simulink model "LV_grid"  (R2021b)
settings: Solver=VariableStepAuto  StartTime=0  StopTime=5.0005  FixedStep=5e-4  RelTol=1e-3
model workspace (MAT data in the model file):
  P2_1 = 3450
  idx = 1
  time_counter = 1
libraries: spsGroundLib x97, spsStairGeneratorLib x96, spsPiSectionLineLib x90, spsThreePhasePISectionLineLib x90, spsVariableInductorLib x48, spsVariableResistorLib x48, spsRMSLib x36, spsThreePhaseVIMeasurementLib x34, spsACVoltageSourceLib x5, spsLinearTransformerLib x5, spsPower3phInstantaneousLib x1, spsThreePhaseMutualInductanceZ1Z0Lib x1
(part 2 of 6)

== system LV_grid/B16 ==
  MATLAB Function : MATLAB Function  TreatAsAtomicUnit=on
  RMS : spsRMSLib/RMS  TrueRMS=on  Freq=50  RMSInit=1  Ts=5e-4
  Three-Phase V-I Measurement : spsThreePhaseVIMeasurementLib/Three-Phase V-I Measurement  VoltageMeasurement=phase-to-ground  SetLabelV=off  LabelV=Vabc_B1  Vpu=on  VpuLL=off  CurrentMeasurement=no  SetLabelI=off  LabelI=Iabc  Ipu=off  Pbase=100e6  Vbase=400/sqrt(2)  OutputType=Complex  PhasorSimulation=off  PSBequivalent=0
  A : PMIOPort  Side=Left
  B : PMIOPort  Port=2  Side=Left
  C : PMIOPort  Port=3  Side=Left
  "N " : PMIOPort  Tag=PMCPort  Port=4  Side=Left
  a : PMIOPort  Tag=PMCPort  Port=5  Side=Right
  b : PMIOPort  Tag=PMCPort  Port=6  Side=Right
  c : PMIOPort  Tag=PMCPort  Port=7  Side=Right
  n : PMIOPort  Tag=PMCPort  Port=8  Side=Right
  V_out : Outport
  tag scope: Vabc_B16=global
  wires:
  Three-Phase V-I Measurement/1 -> RMS/1
  RMS/1 -> MATLAB Function/1(u)
  MATLAB Function/1(y) -> [Vabc_B16], V_out/1
  connections:
  A/RConn1 -- Three-Phase V-I Measurement/LConn1
  B/RConn1 -- Three-Phase V-I Measurement/LConn2
  C/RConn1 -- Three-Phase V-I Measurement/LConn3
  a/RConn1 -- Three-Phase V-I Measurement/RConn1
  b/RConn1 -- Three-Phase V-I Measurement/RConn2
  c/RConn1 -- Three-Phase V-I Measurement/RConn3
  n/RConn1 -- "N "/RConn1

== system LV_grid/B17 ==
  MATLAB Function : MATLAB Function  TreatAsAtomicUnit=on
  RMS : spsRMSLib/RMS  TrueRMS=on  Freq=50  RMSInit=1  Ts=5e-4
  Three-Phase V-I Measurement : spsThreePhaseVIMeasurementLib/Three-Phase V-I Measurement  VoltageMeasurement=phase-to-ground  SetLabelV=off  LabelV=Vabc_B1  Vpu=on  VpuLL=off  CurrentMeasurement=no  SetLabelI=off  LabelI=Iabc  Ipu=off  Pbase=100e6  Vbase=400/sqrt(2)  OutputType=Complex  PhasorSimulation=off  PSBequivalent=0
  A : PMIOPort  Side=Left
  B : PMIOPort  Port=2  Side=Left
  C : PMIOPort  Port=3  Side=Left
  "N " : PMIOPort  Tag=PMCPort  Port=4  Side=Left
  a : PMIOPort  Tag=PMCPort  Port=5  Side=Right
  b : PMIOPort  Tag=PMCPort  Port=6  Side=Right
  c : PMIOPort  Tag=PMCPort  Port=7  Side=Right
  n : PMIOPort  Tag=PMCPort  Port=8  Side=Right
  V_out : Outport
  tag scope: Vabc_B17=global
  wires:
  Three-Phase V-I Measurement/1 -> RMS/1
  RMS/1 -> MATLAB Function/1(u)
  MATLAB Function/1(y) -> [Vabc_B17], V_out/1
  connections:
  A/RConn1 -- Three-Phase V-I Measurement/LConn1
  B/RConn1 -- Three-Phase V-I Measurement/LConn2
  C/RConn1 -- Three-Phase V-I Measurement/LConn3
  a/RConn1 -- Three-Phase V-I Measurement/RConn1
  b/RConn1 -- Three-Phase V-I Measurement/RConn2
  c/RConn1 -- Three-Phase V-I Measurement/RConn3
  n/RConn1 -- "N "/RConn1

== system LV_grid/B18 ==
  MATLAB Function : MATLAB Function  TreatAsAtomicUnit=on
  RMS : spsRMSLib/RMS  TrueRMS=on  Freq=50  RMSInit=1  Ts=5e-4
  Three-Phase V-I Measurement : spsThreePhaseVIMeasurementLib/Three-Phase V-I Measurement  VoltageMeasurement=phase-to-ground  SetLabelV=off  LabelV=Vabc_B1  Vpu=on  VpuLL=off  CurrentMeasurement=no  SetLabelI=off  LabelI=Iabc  Ipu=off  Pbase=100e6  Vbase=400/sqrt(2)  OutputType=Complex  PhasorSimulation=off  PSBequivalent=0
  A : PMIOPort  Side=Left
  B : PMIOPort  Port=2  Side=Left
  C : PMIOPort  Port=3  Side=Left
  "N " : PMIOPort  Tag=PMCPort  Port=4  Side=Left
  a : PMIOPort  Tag=PMCPort  Port=5  Side=Right
  b : PMIOPort  Tag=PMCPort  Port=6  Side=Right
  c : PMIOPort  Tag=PMCPort  Port=7  Side=Right
  n : PMIOPort  Tag=PMCPort  Port=8  Side=Right
  V_out : Outport
  tag scope: Vabc_B18=global
  wires:
  Three-Phase V-I Measurement/1 -> RMS/1
  RMS/1 -> MATLAB Function/1(u)
  MATLAB Function/1(y) -> [Vabc_B18], V_out/1
  connections:
  A/RConn1 -- Three-Phase V-I Measurement/LConn1
  B/RConn1 -- Three-Phase V-I Measurement/LConn2
  C/RConn1 -- Three-Phase V-I Measurement/LConn3
  a/RConn1 -- Three-Phase V-I Measurement/RConn1
  b/RConn1 -- Three-Phase V-I Measurement/RConn2
  c/RConn1 -- Three-Phase V-I Measurement/RConn3
  n/RConn1 -- "N "/RConn1

== system LV_grid/B19 ==
  MATLAB Function : MATLAB Function  TreatAsAtomicUnit=on
  RMS : spsRMSLib/RMS  TrueRMS=on  Freq=50  RMSInit=1  Ts=5e-4
  Three-Phase V-I Measurement : spsThreePhaseVIMeasurementLib/Three-Phase V-I Measurement  VoltageMeasurement=phase-to-ground  SetLabelV=off  LabelV=Vabc_B1  Vpu=on  VpuLL=off  CurrentMeasurement=no  SetLabelI=off  LabelI=Iabc  Ipu=off  Pbase=100e6  Vbase=400/sqrt(2)  OutputType=Complex  PhasorSimulation=off  PSBequivalent=0
  A : PMIOPort  Side=Left
  B : PMIOPort  Port=2  Side=Left
  C : PMIOPort  Port=3  Side=Left
  "N " : PMIOPort  Tag=PMCPort  Port=4  Side=Left
  a : PMIOPort  Tag=PMCPort  Port=5  Side=Right
  b : PMIOPort  Tag=PMCPort  Port=6  Side=Right
  c : PMIOPort  Tag=PMCPort  Port=7  Side=Right
  n : PMIOPort  Tag=PMCPort  Port=8  Side=Right
  V_out : Outport
  tag scope: Vabc_B19=global
  wires:
  Three-Phase V-I Measurement/1 -> RMS/1
  MATLAB Function/1(y) -> [Vabc_B19], V_out/1
  RMS/1 -> MATLAB Function/1(u)
  connections:
  A/RConn1 -- Three-Phase V-I Measurement/LConn1
  B/RConn1 -- Three-Phase V-I Measurement/LConn2
  C/RConn1 -- Three-Phase V-I Measurement/LConn3
  a/RConn1 -- Three-Phase V-I Measurement/RConn1
  b/RConn1 -- Three-Phase V-I Measurement/RConn2
  c/RConn1 -- Three-Phase V-I Measurement/RConn3
  n/RConn1 -- "N "/RConn1

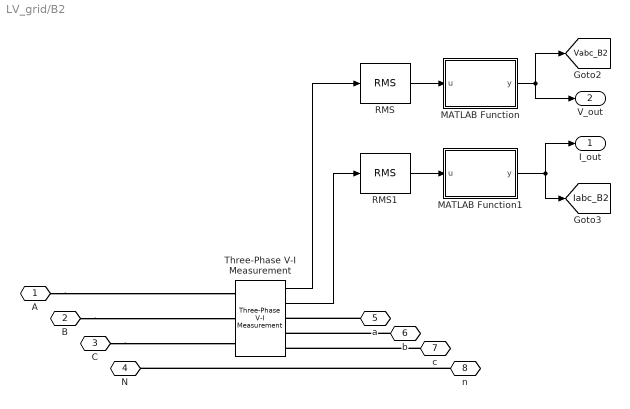
== system LV_grid/B2 ==
  MATLAB Function : MATLAB Function  TreatAsAtomicUnit=on
  MATLAB Function1 : MATLAB Function  TreatAsAtomicUnit=on
  RMS : spsRMSLib/RMS  TrueRMS=on  Freq=50  RMSInit=1  Ts=5e-4
  RMS1 : spsRMSLib/RMS  TrueRMS=on  Freq=50  RMSInit=1  Ts=5e-4
  Three-Phase V-I Measurement : spsThreePhaseVIMeasurementLib/Three-Phase V-I Measurement  VoltageMeasurement=phase-to-ground  SetLabelV=off  LabelV=Vabc_B1  Vpu=on  VpuLL=off  CurrentMeasurement=yes  SetLabelI=off  LabelI=Iabc  Ipu=on  Pbase=250e3  Vbase=400/sqrt(2)  OutputType=Magnitude  PhasorSimulation=off  PSBequivalent=0
  A : PMIOPort  Side=Left
  B : PMIOPort  Port=2  Side=Left
  C : PMIOPort  Port=3  Side=Left
  N : PMIOPort  Tag=PMCPort  Port=4  Side=Left
  a : PMIOPort  Tag=PMCPort  Port=5  Side=Right
  b : PMIOPort  Tag=PMCPort  Port=6  Side=Right
  c : PMIOPort  Tag=PMCPort  Port=7  Side=Right
  n : PMIOPort  Tag=PMCPort  Port=8  Side=Right
  I_out : Outport
  V_out : Outport  Port=2
  tag scope: Iabc_B2=global, Vabc_B2=global
  wires:
  Three-Phase V-I Measurement/1 -> RMS/1
  Three-Phase V-I Measurement/2 -> RMS1/1
  MATLAB Function/1(y) -> [Vabc_B2], V_out/1
  RMS/1 -> MATLAB Function/1(u)
  RMS1/1 -> MATLAB Function1/1(u)
  MATLAB Function1/1(y) -> [Iabc_B2], I_out/1
  connections:
  B/RConn1 -- Three-Phase V-I Measurement/LConn2
  n/RConn1 -- N/RConn1
  c/RConn1 -- Three-Phase V-I Measurement/RConn3
  b/RConn1 -- Three-Phase V-I Measurement/RConn2
  C/RConn1 -- Three-Phase V-I Measurement/LConn3
  a/RConn1 -- Three-Phase V-I Measurement/RConn1
  A/RConn1 -- Three-Phase V-I Measurement/LConn1

== system LV_grid/B20 ==
  MATLAB Function : MATLAB Function  TreatAsAtomicUnit=on
  RMS : spsRMSLib/RMS  TrueRMS=on  Freq=50  RMSInit=1  Ts=5e-4
  Three-Phase V-I Measurement : spsThreePhaseVIMeasurementLib/Three-Phase V-I Measurement  VoltageMeasurement=phase-to-ground  SetLabelV=off  LabelV=Vabc_B1  Vpu=on  VpuLL=off  CurrentMeasurement=no  SetLabelI=off  LabelI=Iabc  Ipu=off  Pbase=100e6  Vbase=400/sqrt(2)  OutputType=Complex  PhasorSimulation=off  PSBequivalent=0
  A : PMIOPort  Side=Left
  B : PMIOPort  Port=2  Side=Left
  C : PMIOPort  Port=3  Side=Left
  "N " : PMIOPort  Tag=PMCPort  Port=4  Side=Left
  a : PMIOPort  Tag=PMCPort  Port=5  Side=Right
  b : PMIOPort  Tag=PMCPort  Port=6  Side=Right
  c : PMIOPort  Tag=PMCPort  Port=7  Side=Right
  n : PMIOPort  Tag=PMCPort  Port=8  Side=Right
  V_out : Outport
  tag scope: Vabc_B20=global
  wires:
  Three-Phase V-I Measurement/1 -> RMS/1
  RMS/1 -> MATLAB Function/1(u)
  MATLAB Function/1(y) -> [Vabc_B20], V_out/1
  connections:
  A/RConn1 -- Three-Phase V-I Measurement/LConn1
  B/RConn1 -- Three-Phase V-I Measurement/LConn2
  C/RConn1 -- Three-Phase V-I Measurement/LConn3
  a/RConn1 -- Three-Phase V-I Measurement/RConn1
  b/RConn1 -- Three-Phase V-I Measurement/RConn2
  c/RConn1 -- Three-Phase V-I Measurement/RConn3
  n/RConn1 -- "N "/RConn1

== system LV_grid/B21 ==
  MATLAB Function : MATLAB Function  TreatAsAtomicUnit=on
  RMS : spsRMSLib/RMS  TrueRMS=on  Freq=50  RMSInit=1  Ts=5e-4
  Three-Phase V-I Measurement : spsThreePhaseVIMeasurementLib/Three-Phase V-I Measurement  VoltageMeasurement=phase-to-ground  SetLabelV=off  LabelV=Vabc_B1  Vpu=on  VpuLL=off  CurrentMeasurement=no  SetLabelI=off  LabelI=Iabc  Ipu=off  Pbase=100e6  Vbase=400/sqrt(2)  OutputType=Complex  PhasorSimulation=off  PSBequivalent=0
  A : PMIOPort  Side=Left
  B : PMIOPort  Port=2  Side=Left
  C : PMIOPort  Port=3  Side=Left
  "N " : PMIOPort  Tag=PMCPort  Port=4  Side=Left
  a : PMIOPort  Tag=PMCPort  Port=5  Side=Right
  b : PMIOPort  Tag=PMCPort  Port=6  Side=Right
  c : PMIOPort  Tag=PMCPort  Port=7  Side=Right
  n : PMIOPort  Tag=PMCPort  Port=8  Side=Right
  V_out : Outport
  tag scope: Vabc_B21=global
  wires:
  Three-Phase V-I Measurement/1 -> RMS/1
  RMS/1 -> MATLAB Function/1(u)
  MATLAB Function/1(y) -> [Vabc_B21], V_out/1
  connections:
  A/RConn1 -- Three-Phase V-I Measurement/LConn1
  B/RConn1 -- Three-Phase V-I Measurement/LConn2
  C/RConn1 -- Three-Phase V-I Measurement/LConn3
  a/RConn1 -- Three-Phase V-I Measurement/RConn1
  b/RConn1 -- Three-Phase V-I Measurement/RConn2
  c/RConn1 -- Three-Phase V-I Measurement/RConn3
  n/RConn1 -- "N "/RConn1

== system LV_grid/B22 ==
  MATLAB Function : MATLAB Function  TreatAsAtomicUnit=on
  RMS : spsRMSLib/RMS  TrueRMS=on  Freq=50  RMSInit=1  Ts=5e-4
  Three-Phase V-I Measurement : spsThreePhaseVIMeasurementLib/Three-Phase V-I Measurement  VoltageMeasurement=phase-to-ground  SetLabelV=off  LabelV=Vabc_B1  Vpu=on  VpuLL=off  CurrentMeasurement=no  SetLabelI=off  LabelI=Iabc  Ipu=off  Pbase=100e6  Vbase=400/sqrt(2)  OutputType=Complex  PhasorSimulation=off  PSBequivalent=0
  A : PMIOPort  Side=Left
  B : PMIOPort  Port=2  Side=Left
  C : PMIOPort  Port=3  Side=Left
  "N " : PMIOPort  Tag=PMCPort  Port=4  Side=Left
  a : PMIOPort  Tag=PMCPort  Port=5  Side=Right
  b : PMIOPort  Tag=PMCPort  Port=6  Side=Right
  c : PMIOPort  Tag=PMCPort  Port=7  Side=Right
  n : PMIOPort  Tag=PMCPort  Port=8  Side=Right
  V_out : Outport
  tag scope: Vabc_B22=global
  wires:
  Three-Phase V-I Measurement/1 -> RMS/1
  RMS/1 -> MATLAB Function/1(u)
  MATLAB Function/1(y) -> [Vabc_B22], V_out/1
  connections:
  A/RConn1 -- Three-Phase V-I Measurement/LConn1
  B/RConn1 -- Three-Phase V-I Measurement/LConn2
  C/RConn1 -- Three-Phase V-I Measurement/LConn3
  a/RConn1 -- Three-Phase V-I Measurement/RConn1
  b/RConn1 -- Three-Phase V-I Measurement/RConn2
  c/RConn1 -- Three-Phase V-I Measurement/RConn3
  n/RConn1 -- "N "/RConn1

== system LV_grid/B23 ==
  MATLAB Function : MATLAB Function  TreatAsAtomicUnit=on
  RMS : spsRMSLib/RMS  TrueRMS=on  Freq=50  RMSInit=1  Ts=5e-4
  Three-Phase V-I Measurement : spsThreePhaseVIMeasurementLib/Three-Phase V-I Measurement  VoltageMeasurement=phase-to-ground  SetLabelV=off  LabelV=Vabc_B1  Vpu=on  VpuLL=off  CurrentMeasurement=no  SetLabelI=off  LabelI=Iabc  Ipu=off  Pbase=100e6  Vbase=400/sqrt(2)  OutputType=Complex  PhasorSimulation=off  PSBequivalent=0
  A : PMIOPort  Side=Left
  B : PMIOPort  Port=2  Side=Left
  C : PMIOPort  Port=3  Side=Left
  "N " : PMIOPort  Tag=PMCPort  Port=4  Side=Left
  a : PMIOPort  Tag=PMCPort  Port=5  Side=Right
  b : PMIOPort  Tag=PMCPort  Port=6  Side=Right
  c : PMIOPort  Tag=PMCPort  Port=7  Side=Right
  n : PMIOPort  Tag=PMCPort  Port=8  Side=Right
  V_out : Outport
  tag scope: Vabc_B23=global
  wires:
  Three-Phase V-I Measurement/1 -> RMS/1
  RMS/1 -> MATLAB Function/1(u)
  MATLAB Function/1(y) -> [Vabc_B23], V_out/1
  connections:
  A/RConn1 -- Three-Phase V-I Measurement/LConn1
  B/RConn1 -- Three-Phase V-I Measurement/LConn2
  C/RConn1 -- Three-Phase V-I Measurement/LConn3
  a/RConn1 -- Three-Phase V-I Measurement/RConn1
  b/RConn1 -- Three-Phase V-I Measurement/RConn2
  c/RConn1 -- Three-Phase V-I Measurement/RConn3
  n/RConn1 -- "N "/RConn1

== system LV_grid/B24 ==
  MATLAB Function : MATLAB Function  TreatAsAtomicUnit=on
  RMS : spsRMSLib/RMS  TrueRMS=on  Freq=50  RMSInit=1  Ts=5e-4
  Three-Phase V-I Measurement : spsThreePhaseVIMeasurementLib/Three-Phase V-I Measurement  VoltageMeasurement=phase-to-ground  SetLabelV=off  LabelV=Vabc_B1  Vpu=on  VpuLL=off  CurrentMeasurement=no  SetLabelI=off  LabelI=Iabc  Ipu=off  Pbase=100e6  Vbase=400/sqrt(2)  OutputType=Complex  PhasorSimulation=off  PSBequivalent=0
  A : PMIOPort  Side=Left
  B : PMIOPort  Port=2  Side=Left
  C : PMIOPort  Port=3  Side=Left
  "N " : PMIOPort  Tag=PMCPort  Port=4  Side=Left
  a : PMIOPort  Tag=PMCPort  Port=5  Side=Right
  b : PMIOPort  Tag=PMCPort  Port=6  Side=Right
  c : PMIOPort  Tag=PMCPort  Port=7  Side=Right
  n : PMIOPort  Tag=PMCPort  Port=8  Side=Right
  V_out : Outport
  tag scope: Vabc_B24=global
  wires:
  Three-Phase V-I Measurement/1 -> RMS/1
  RMS/1 -> MATLAB Function/1(u)
  MATLAB Function/1(y) -> [Vabc_B24], V_out/1
  connections:
  A/RConn1 -- Three-Phase V-I Measurement/LConn1
  B/RConn1 -- Three-Phase V-I Measurement/LConn2
  C/RConn1 -- Three-Phase V-I Measurement/LConn3
  a/RConn1 -- Three-Phase V-I Measurement/RConn1
  b/RConn1 -- Three-Phase V-I Measurement/RConn2
  c/RConn1 -- Three-Phase V-I Measurement/RConn3
  n/RConn1 -- "N "/RConn1

== system LV_grid/B25 ==
  MATLAB Function : MATLAB Function  TreatAsAtomicUnit=on
  RMS : spsRMSLib/RMS  TrueRMS=on  Freq=50  RMSInit=1  Ts=5e-4
  Three-Phase V-I Measurement : spsThreePhaseVIMeasurementLib/Three-Phase V-I Measurement  VoltageMeasurement=phase-to-ground  SetLabelV=off  LabelV=Vabc_B1  Vpu=on  VpuLL=off  CurrentMeasurement=no  SetLabelI=off  LabelI=Iabc  Ipu=off  Pbase=100e6  Vbase=400/sqrt(2)  OutputType=Complex  PhasorSimulation=off  PSBequivalent=0
  A : PMIOPort  Side=Left
  B : PMIOPort  Port=2  Side=Left
  C : PMIOPort  Port=3  Side=Left
  "N " : PMIOPort  Tag=PMCPort  Port=4  Side=Left
  a : PMIOPort  Tag=PMCPort  Port=5  Side=Right
  b : PMIOPort  Tag=PMCPort  Port=6  Side=Right
  c : PMIOPort  Tag=PMCPort  Port=7  Side=Right
  n : PMIOPort  Tag=PMCPort  Port=8  Side=Right
  V_out : Outport
  tag scope: Vabc_B25=global
  wires:
  Three-Phase V-I Measurement/1 -> RMS/1
  RMS/1 -> MATLAB Function/1(u)
  MATLAB Function/1(y) -> [Vabc_B25], V_out/1
  connections:
  A/RConn1 -- Three-Phase V-I Measurement/LConn1
  B/RConn1 -- Three-Phase V-I Measurement/LConn2
  C/RConn1 -- Three-Phase V-I Measurement/LConn3
  a/RConn1 -- Three-Phase V-I Measurement/RConn1
  b/RConn1 -- Three-Phase V-I Measurement/RConn2
  c/RConn1 -- Three-Phase V-I Measurement/RConn3
  n/RConn1 -- "N "/RConn1

== system LV_grid/B26 ==
  MATLAB Function : MATLAB Function  TreatAsAtomicUnit=on
  RMS : spsRMSLib/RMS  TrueRMS=on  Freq=50  RMSInit=1  Ts=5e-4
  Three-Phase V-I Measurement : spsThreePhaseVIMeasurementLib/Three-Phase V-I Measurement  VoltageMeasurement=phase-to-ground  SetLabelV=off  LabelV=Vabc_B1  Vpu=on  VpuLL=off  CurrentMeasurement=no  SetLabelI=off  LabelI=Iabc  Ipu=off  Pbase=100e6  Vbase=400/sqrt(2)  OutputType=Complex  PhasorSimulation=off  PSBequivalent=0
  A : PMIOPort  Side=Left
  B : PMIOPort  Port=2  Side=Left
  C : PMIOPort  Port=3  Side=Left
  "N " : PMIOPort  Tag=PMCPort  Port=4  Side=Left
  a : PMIOPort  Tag=PMCPort  Port=5  Side=Right
  b : PMIOPort  Tag=PMCPort  Port=6  Side=Right
  c : PMIOPort  Tag=PMCPort  Port=7  Side=Right
  n : PMIOPort  Tag=PMCPort  Port=8  Side=Right
  V_out : Outport
  tag scope: Vabc_B26=global
  wires:
  Three-Phase V-I Measurement/1 -> RMS/1
  RMS/1 -> MATLAB Function/1(u)
  MATLAB Function/1(y) -> [Vabc_B26], V_out/1
  connections:
  A/RConn1 -- Three-Phase V-I Measurement/LConn1
  B/RConn1 -- Three-Phase V-I Measurement/LConn2
  C/RConn1 -- Three-Phase V-I Measurement/LConn3
  a/RConn1 -- Three-Phase V-I Measurement/RConn1
  b/RConn1 -- Three-Phase V-I Measurement/RConn2
  c/RConn1 -- Three-Phase V-I Measurement/RConn3
  n/RConn1 -- "N "/RConn1

== system LV_grid/B27 ==
  MATLAB Function : MATLAB Function  TreatAsAtomicUnit=on
  RMS : spsRMSLib/RMS  TrueRMS=on  Freq=50  RMSInit=1  Ts=5e-4
  Three-Phase V-I Measurement : spsThreePhaseVIMeasurementLib/Three-Phase V-I Measurement  VoltageMeasurement=phase-to-ground  SetLabelV=off  LabelV=Vabc_B1  Vpu=on  VpuLL=off  CurrentMeasurement=no  SetLabelI=off  LabelI=Iabc  Ipu=off  Pbase=100e6  Vbase=400/sqrt(2)  OutputType=Complex  PhasorSimulation=off  PSBequivalent=0
  A : PMIOPort  Side=Left
  B : PMIOPort  Port=2  Side=Left
  C : PMIOPort  Port=3  Side=Left
  "N " : PMIOPort  Tag=PMCPort  Port=4  Side=Left
  a : PMIOPort  Tag=PMCPort  Port=5  Side=Right
  b : PMIOPort  Tag=PMCPort  Port=6  Side=Right
  c : PMIOPort  Tag=PMCPort  Port=7  Side=Right
  n : PMIOPort  Tag=PMCPort  Port=8  Side=Right
  V_out : Outport
  tag scope: Vabc_B27=global
  wires:
  Three-Phase V-I Measurement/1 -> RMS/1
  RMS/1 -> MATLAB Function/1(u)
  MATLAB Function/1(y) -> [Vabc_B27], V_out/1
  connections:
  A/RConn1 -- Three-Phase V-I Measurement/LConn1
  B/RConn1 -- Three-Phase V-I Measurement/LConn2
  C/RConn1 -- Three-Phase V-I Measurement/LConn3
  a/RConn1 -- Three-Phase V-I Measurement/RConn1
  b/RConn1 -- Three-Phase V-I Measurement/RConn2
  c/RConn1 -- Three-Phase V-I Measurement/RConn3
  n/RConn1 -- "N "/RConn1

== system LV_grid/B28 ==
  MATLAB Function : MATLAB Function  TreatAsAtomicUnit=on
  RMS : spsRMSLib/RMS  TrueRMS=on  Freq=50  RMSInit=1  Ts=5e-4
  Three-Phase V-I Measurement : spsThreePhaseVIMeasurementLib/Three-Phase V-I Measurement  VoltageMeasurement=phase-to-ground  SetLabelV=off  LabelV=Vabc_B1  Vpu=on  VpuLL=off  CurrentMeasurement=no  SetLabelI=off  LabelI=Iabc  Ipu=off  Pbase=100e6  Vbase=400/sqrt(2)  OutputType=Complex  PhasorSimulation=off  PSBequivalent=0
  A : PMIOPort  Side=Left
  B : PMIOPort  Port=2  Side=Left
  C : PMIOPort  Port=3  Side=Left
  "N " : PMIOPort  Tag=PMCPort  Port=4  Side=Left
  a : PMIOPort  Tag=PMCPort  Port=5  Side=Right
  b : PMIOPort  Tag=PMCPort  Port=6  Side=Right
  c : PMIOPort  Tag=PMCPort  Port=7  Side=Right
  n : PMIOPort  Tag=PMCPort  Port=8  Side=Right
  V_out : Outport
  tag scope: Vabc_B28=global
  wires:
  Three-Phase V-I Measurement/1 -> RMS/1
  RMS/1 -> MATLAB Function/1(u)
  MATLAB Function/1(y) -> [Vabc_B28], V_out/1
  connections:
  A/RConn1 -- Three-Phase V-I Measurement/LConn1
  B/RConn1 -- Three-Phase V-I Measurement/LConn2
  C/RConn1 -- Three-Phase V-I Measurement/LConn3
  a/RConn1 -- Three-Phase V-I Measurement/RConn1
  b/RConn1 -- Three-Phase V-I Measurement/RConn2
  c/RConn1 -- Three-Phase V-I Measurement/RConn3
  n/RConn1 -- "N "/RConn1

== system LV_grid/B29 ==
  MATLAB Function : MATLAB Function  TreatAsAtomicUnit=on
  RMS : spsRMSLib/RMS  TrueRMS=on  Freq=50  RMSInit=1  Ts=5e-4
  Three-Phase V-I Measurement : spsThreePhaseVIMeasurementLib/Three-Phase V-I Measurement  VoltageMeasurement=phase-to-ground  SetLabelV=off  LabelV=Vabc_B1  Vpu=on  VpuLL=off  CurrentMeasurement=no  SetLabelI=off  LabelI=Iabc  Ipu=off  Pbase=100e6  Vbase=400/sqrt(2)  OutputType=Complex  PhasorSimulation=off  PSBequivalent=0
  A : PMIOPort  Side=Left
  B : PMIOPort  Port=2  Side=Left
  C : PMIOPort  Port=3  Side=Left
  "N " : PMIOPort  Tag=PMCPort  Port=4  Side=Left
  a : PMIOPort  Tag=PMCPort  Port=5  Side=Right
  b : PMIOPort  Tag=PMCPort  Port=6  Side=Right
  c : PMIOPort  Tag=PMCPort  Port=7  Side=Right
  n : PMIOPort  Tag=PMCPort  Port=8  Side=Right
  V_out : Outport
  tag scope: Vabc_B29=global
  wires:
  Three-Phase V-I Measurement/1 -> RMS/1
  RMS/1 -> MATLAB Function/1(u)
  MATLAB Function/1(y) -> [Vabc_B29], V_out/1
  connections:
  A/RConn1 -- Three-Phase V-I Measurement/LConn1
  B/RConn1 -- Three-Phase V-I Measurement/LConn2
  C/RConn1 -- Three-Phase V-I Measurement/LConn3
  a/RConn1 -- Three-Phase V-I Measurement/RConn1
  b/RConn1 -- Three-Phase V-I Measurement/RConn2
  c/RConn1 -- Three-Phase V-I Measurement/RConn3
  n/RConn1 -- "N "/RConn1

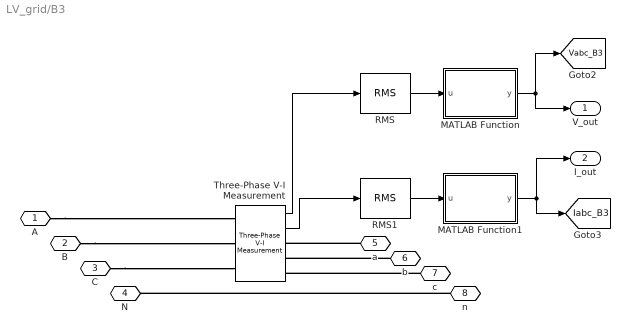
== system LV_grid/B3 ==
  MATLAB Function : MATLAB Function  TreatAsAtomicUnit=on
  MATLAB Function1 : MATLAB Function  TreatAsAtomicUnit=on
  RMS : spsRMSLib/RMS  TrueRMS=on  Freq=50  RMSInit=1  Ts=5e-4
  RMS1 : spsRMSLib/RMS  TrueRMS=on  Freq=50  RMSInit=1  Ts=5e-4
  Three-Phase V-I Measurement : spsThreePhaseVIMeasurementLib/Three-Phase V-I Measurement  VoltageMeasurement=phase-to-ground  SetLabelV=off  LabelV=Vabc_B1  Vpu=on  VpuLL=off  CurrentMeasurement=yes  SetLabelI=off  LabelI=Iabc  Ipu=on  Pbase=250e3  Vbase=400/sqrt(2)  OutputType=Magnitude  PhasorSimulation=off  PSBequivalent=0
  A : PMIOPort  Side=Left
  B : PMIOPort  Port=2  Side=Left
  C : PMIOPort  Port=3  Side=Left
  N : PMIOPort  Tag=PMCPort  Port=4  Side=Left
  a : PMIOPort  Tag=PMCPort  Port=5  Side=Right
  b : PMIOPort  Tag=PMCPort  Port=6  Side=Right
  c : PMIOPort  Tag=PMCPort  Port=7  Side=Right
  n : PMIOPort  Tag=PMCPort  Port=8  Side=Right
  V_out : Outport
  I_out : Outport  Port=2
  tag scope: Iabc_B3=global, Vabc_B3=global
  wires:
  Three-Phase V-I Measurement/2 -> RMS1/1
  RMS/1 -> MATLAB Function/1(u)
  MATLAB Function/1(y) -> V_out/1, [Vabc_B3]
  Three-Phase V-I Measurement/1 -> RMS/1
  MATLAB Function1/1(y) -> [Iabc_B3], I_out/1
  RMS1/1 -> MATLAB Function1/1(u)
  connections:
  B/RConn1 -- Three-Phase V-I Measurement/LConn2
  n/RConn1 -- N/RConn1
  c/RConn1 -- Three-Phase V-I Measurement/RConn3
  b/RConn1 -- Three-Phase V-I Measurement/RConn2
  C/RConn1 -- Three-Phase V-I Measurement/LConn3
  a/RConn1 -- Three-Phase V-I Measurement/RConn1
  A/RConn1 -- Three-Phase V-I Measurement/LConn1

== system LV_grid/B30 ==
  MATLAB Function : MATLAB Function  TreatAsAtomicUnit=on
  RMS : spsRMSLib/RMS  TrueRMS=on  Freq=50  RMSInit=1  Ts=5e-4
  Three-Phase V-I Measurement : spsThreePhaseVIMeasurementLib/Three-Phase V-I Measurement  VoltageMeasurement=phase-to-ground  SetLabelV=off  LabelV=Vabc_B1  Vpu=on  VpuLL=off  CurrentMeasurement=no  SetLabelI=off  LabelI=Iabc  Ipu=off  Pbase=100e6  Vbase=400/sqrt(2)  OutputType=Complex  PhasorSimulation=off  PSBequivalent=0
  A : PMIOPort  Side=Left
  B : PMIOPort  Port=2  Side=Left
  C : PMIOPort  Port=3  Side=Left
  "N " : PMIOPort  Tag=PMCPort  Port=4  Side=Left
  a : PMIOPort  Tag=PMCPort  Port=5  Side=Right
  b : PMIOPort  Tag=PMCPort  Port=6  Side=Right
  c : PMIOPort  Tag=PMCPort  Port=7  Side=Right
  n : PMIOPort  Tag=PMCPort  Port=8  Side=Right
  V_out : Outport
  tag scope: Vabc_B30=global
  wires:
  Three-Phase V-I Measurement/1 -> RMS/1
  MATLAB Function/1(y) -> [Vabc_B30], V_out/1
  RMS/1 -> MATLAB Function/1(u)
  connections:
  A/RConn1 -- Three-Phase V-I Measurement/LConn1
  B/RConn1 -- Three-Phase V-I Measurement/LConn2
  C/RConn1 -- Three-Phase V-I Measurement/LConn3
  a/RConn1 -- Three-Phase V-I Measurement/RConn1
  b/RConn1 -- Three-Phase V-I Measurement/RConn2
  c/RConn1 -- Three-Phase V-I Measurement/RConn3
  n/RConn1 -- "N "/RConn1

== system LV_grid/B31 ==
  MATLAB Function : MATLAB Function  TreatAsAtomicUnit=on
  RMS : spsRMSLib/RMS  TrueRMS=on  Freq=50  RMSInit=1  Ts=5e-4
  Three-Phase V-I Measurement : spsThreePhaseVIMeasurementLib/Three-Phase V-I Measurement  VoltageMeasurement=phase-to-ground  SetLabelV=off  LabelV=Vabc_B1  Vpu=on  VpuLL=off  CurrentMeasurement=no  SetLabelI=off  LabelI=Iabc  Ipu=off  Pbase=100e6  Vbase=400/sqrt(2)  OutputType=Complex  PhasorSimulation=off  PSBequivalent=0
  A : PMIOPort  Side=Left
  B : PMIOPort  Port=2  Side=Left
  C : PMIOPort  Port=3  Side=Left
  "N " : PMIOPort  Tag=PMCPort  Port=4  Side=Left
  a : PMIOPort  Tag=PMCPort  Port=5  Side=Right
  b : PMIOPort  Tag=PMCPort  Port=6  Side=Right
  c : PMIOPort  Tag=PMCPort  Port=7  Side=Right
  n : PMIOPort  Tag=PMCPort  Port=8  Side=Right
  V_out : Outport
  tag scope: Vabc_B31=global
  wires:
  Three-Phase V-I Measurement/1 -> RMS/1
  RMS/1 -> MATLAB Function/1(u)
  MATLAB Function/1(y) -> [Vabc_B31], V_out/1
  connections:
  A/RConn1 -- Three-Phase V-I Measurement/LConn1
  B/RConn1 -- Three-Phase V-I Measurement/LConn2
  C/RConn1 -- Three-Phase V-I Measurement/LConn3
  a/RConn1 -- Three-Phase V-I Measurement/RConn1
  b/RConn1 -- Three-Phase V-I Measurement/RConn2
  c/RConn1 -- Three-Phase V-I Measurement/RConn3
  n/RConn1 -- "N "/RConn1

== system LV_grid/B32 ==
  MATLAB Function : MATLAB Function  TreatAsAtomicUnit=on
  RMS : spsRMSLib/RMS  TrueRMS=on  Freq=50  RMSInit=1  Ts=5e-4
  Three-Phase V-I Measurement : spsThreePhaseVIMeasurementLib/Three-Phase V-I Measurement  VoltageMeasurement=phase-to-ground  SetLabelV=off  LabelV=Vabc_B1  Vpu=on  VpuLL=off  CurrentMeasurement=no  SetLabelI=off  LabelI=Iabc  Ipu=off  Pbase=100e6  Vbase=400/sqrt(2)  OutputType=Complex  PhasorSimulation=off  PSBequivalent=0
  A : PMIOPort  Side=Left
  B : PMIOPort  Port=2  Side=Left
  C : PMIOPort  Port=3  Side=Left
  "N " : PMIOPort  Tag=PMCPort  Port=4  Side=Left
  a : PMIOPort  Tag=PMCPort  Port=5  Side=Right
  b : PMIOPort  Tag=PMCPort  Port=6  Side=Right
  c : PMIOPort  Tag=PMCPort  Port=7  Side=Right
  n : PMIOPort  Tag=PMCPort  Port=8  Side=Right
  V_out : Outport
  tag scope: Vabc_B32=global
  wires:
  Three-Phase V-I Measurement/1 -> RMS/1
  RMS/1 -> MATLAB Function/1(u)
  MATLAB Function/1(y) -> [Vabc_B32], V_out/1
  connections:
  A/RConn1 -- Three-Phase V-I Measurement/LConn1
  B/RConn1 -- Three-Phase V-I Measurement/LConn2
  C/RConn1 -- Three-Phase V-I Measurement/LConn3
  a/RConn1 -- Three-Phase V-I Measurement/RConn1
  b/RConn1 -- Three-Phase V-I Measurement/RConn2
  c/RConn1 -- Three-Phase V-I Measurement/RConn3
  n/RConn1 -- "N "/RConn1

== system LV_grid/B33 ==
  MATLAB Function : MATLAB Function  TreatAsAtomicUnit=on
  RMS : spsRMSLib/RMS  TrueRMS=on  Freq=50  RMSInit=1  Ts=5e-4
  Three-Phase V-I Measurement : spsThreePhaseVIMeasurementLib/Three-Phase V-I Measurement  VoltageMeasurement=phase-to-ground  SetLabelV=off  LabelV=Vabc_B1  Vpu=on  VpuLL=off  CurrentMeasurement=no  SetLabelI=off  LabelI=Iabc  Ipu=off  Pbase=100e6  Vbase=400/sqrt(2)  OutputType=Complex  PhasorSimulation=off  PSBequivalent=0
  A : PMIOPort  Side=Left
  B : PMIOPort  Port=2  Side=Left
  C : PMIOPort  Port=3  Side=Left
  "N " : PMIOPort  Tag=PMCPort  Port=4  Side=Left
  a : PMIOPort  Tag=PMCPort  Port=5  Side=Right
  b : PMIOPort  Tag=PMCPort  Port=6  Side=Right
  c : PMIOPort  Tag=PMCPort  Port=7  Side=Right
  n : PMIOPort  Tag=PMCPort  Port=8  Side=Right
  V_out : Outport
  tag scope: Vabc_B33=global
  wires:
  Three-Phase V-I Measurement/1 -> RMS/1
  RMS/1 -> MATLAB Function/1(u)
  MATLAB Function/1(y) -> [Vabc_B33], V_out/1
  connections:
  A/RConn1 -- Three-Phase V-I Measurement/LConn1
  B/RConn1 -- Three-Phase V-I Measurement/LConn2
  C/RConn1 -- Three-Phase V-I Measurement/LConn3
  a/RConn1 -- Three-Phase V-I Measurement/RConn1
  b/RConn1 -- Three-Phase V-I Measurement/RConn2
  c/RConn1 -- Three-Phase V-I Measurement/RConn3
  n/RConn1 -- "N "/RConn1

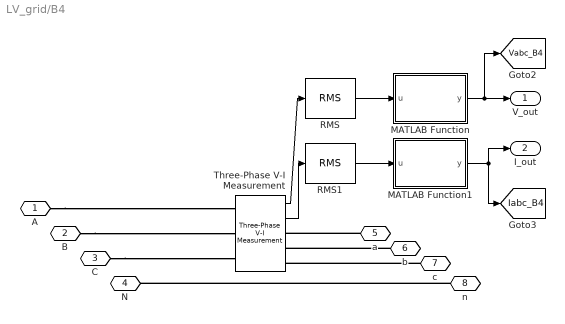
== system LV_grid/B4 ==
  MATLAB Function : MATLAB Function  TreatAsAtomicUnit=on
  MATLAB Function1 : MATLAB Function  TreatAsAtomicUnit=on
  RMS : spsRMSLib/RMS  TrueRMS=on  Freq=50  RMSInit=1  Ts=5e-4
  RMS1 : spsRMSLib/RMS  TrueRMS=on  Freq=50  RMSInit=1  Ts=5e-4
  Three-Phase V-I Measurement : spsThreePhaseVIMeasurementLib/Three-Phase V-I Measurement  VoltageMeasurement=phase-to-ground  SetLabelV=off  LabelV=Vabc_B1  Vpu=on  VpuLL=off  CurrentMeasurement=yes  SetLabelI=off  LabelI=Iabc  Ipu=on  Pbase=250e3  Vbase=400/sqrt(2)  OutputType=Magnitude  PhasorSimulation=off  PSBequivalent=0
  A : PMIOPort  Side=Left
  B : PMIOPort  Port=2  Side=Left
  C : PMIOPort  Port=3  Side=Left
  N : PMIOPort  Tag=PMCPort  Port=4  Side=Left
  a : PMIOPort  Tag=PMCPort  Port=5  Side=Right
  b : PMIOPort  Tag=PMCPort  Port=6  Side=Right
  c : PMIOPort  Tag=PMCPort  Port=7  Side=Right
  n : PMIOPort  Tag=PMCPort  Port=8  Side=Right
  V_out : Outport
  I_out : Outport  Port=2
  tag scope: Iabc_B4=global, Vabc_B4=global
  wires:
  Three-Phase V-I Measurement/1 -> RMS/1
  Three-Phase V-I Measurement/2 -> RMS1/1
  RMS1/1 -> MATLAB Function1/1(u)
  RMS/1 -> MATLAB Function/1(u)
  MATLAB Function/1(y) -> [Vabc_B4], V_out/1
  MATLAB Function1/1(y) -> I_out/1, [Iabc_B4]
  connections:
  B/RConn1 -- Three-Phase V-I Measurement/LConn2
  n/RConn1 -- N/RConn1
  c/RConn1 -- Three-Phase V-I Measurement/RConn3
  b/RConn1 -- Three-Phase V-I Measurement/RConn2
  C/RConn1 -- Three-Phase V-I Measurement/LConn3
  a/RConn1 -- Three-Phase V-I Measurement/RConn1
  A/RConn1 -- Three-Phase V-I Measurement/LConn1

== system LV_grid/B5 ==
  MATLAB Function : MATLAB Function  TreatAsAtomicUnit=on
  RMS : spsRMSLib/RMS  TrueRMS=on  Freq=50  RMSInit=1  Ts=5e-4
  Three-Phase V-I Measurement : spsThreePhaseVIMeasurementLib/Three-Phase V-I Measurement  VoltageMeasurement=phase-to-ground  SetLabelV=off  LabelV=Vabc_B1  Vpu=on  VpuLL=off  CurrentMeasurement=no  SetLabelI=off  LabelI=Iabc  Ipu=off  Pbase=100e6  Vbase=400/sqrt(2)  OutputType=Complex  PhasorSimulation=off  PSBequivalent=0
  A : PMIOPort  Side=Left
  B : PMIOPort  Port=2  Side=Left
  C : PMIOPort  Port=3  Side=Left
  "N " : PMIOPort  Tag=PMCPort  Port=4  Side=Left
  a : PMIOPort  Tag=PMCPort  Port=5  Side=Right
  b : PMIOPort  Tag=PMCPort  Port=6  Side=Right
  c : PMIOPort  Tag=PMCPort  Port=7  Side=Right
  n : PMIOPort  Tag=PMCPort  Port=8  Side=Right
  V_out : Outport
  tag scope: Vabc_B5=global
  wires:
  Three-Phase V-I Measurement/1 -> RMS/1
  MATLAB Function/1(y) -> [Vabc_B5], V_out/1
  RMS/1 -> MATLAB Function/1(u)
  connections:
  A/RConn1 -- Three-Phase V-I Measurement/LConn1
  B/RConn1 -- Three-Phase V-I Measurement/LConn2
  C/RConn1 -- Three-Phase V-I Measurement/LConn3
  a/RConn1 -- Three-Phase V-I Measurement/RConn1
  b/RConn1 -- Three-Phase V-I Measurement/RConn2
  c/RConn1 -- Three-Phase V-I Measurement/RConn3
  n/RConn1 -- "N "/RConn1

== system LV_grid/B6 ==
  MATLAB Function : MATLAB Function  TreatAsAtomicUnit=on
  RMS : spsRMSLib/RMS  TrueRMS=on  Freq=50  RMSInit=1  Ts=5e-4
  Three-Phase V-I Measurement : spsThreePhaseVIMeasurementLib/Three-Phase V-I Measurement  VoltageMeasurement=phase-to-ground  SetLabelV=off  LabelV=Vabc_B1  Vpu=on  VpuLL=off  CurrentMeasurement=no  SetLabelI=off  LabelI=Iabc  Ipu=off  Pbase=100e6  Vbase=400/sqrt(2)  OutputType=Complex  PhasorSimulation=off  PSBequivalent=0
  A : PMIOPort  Side=Left
  B : PMIOPort  Port=2  Side=Left
  C : PMIOPort  Port=3  Side=Left
  "N " : PMIOPort  Tag=PMCPort  Port=4  Side=Left
  a : PMIOPort  Tag=PMCPort  Port=5  Side=Right
  b : PMIOPort  Tag=PMCPort  Port=6  Side=Right
  c : PMIOPort  Tag=PMCPort  Port=7  Side=Right
  n : PMIOPort  Tag=PMCPort  Port=8  Side=Right
  V_out : Outport
  tag scope: Vabc_B6=global
  wires:
  Three-Phase V-I Measurement/1 -> RMS/1
  RMS/1 -> MATLAB Function/1(u)
  MATLAB Function/1(y) -> [Vabc_B6], V_out/1
  connections:
  A/RConn1 -- Three-Phase V-I Measurement/LConn1
  B/RConn1 -- Three-Phase V-I Measurement/LConn2
  C/RConn1 -- Three-Phase V-I Measurement/LConn3
  a/RConn1 -- Three-Phase V-I Measurement/RConn1
  b/RConn1 -- Three-Phase V-I Measurement/RConn2
  c/RConn1 -- Three-Phase V-I Measurement/RConn3
  n/RConn1 -- "N "/RConn1

== system LV_grid/B7 ==
  MATLAB Function : MATLAB Function  TreatAsAtomicUnit=on
  RMS : spsRMSLib/RMS  TrueRMS=on  Freq=50  RMSInit=1  Ts=5e-4
  Three-Phase V-I Measurement : spsThreePhaseVIMeasurementLib/Three-Phase V-I Measurement  VoltageMeasurement=phase-to-ground  SetLabelV=off  LabelV=Vabc_B1  Vpu=on  VpuLL=off  CurrentMeasurement=no  SetLabelI=off  LabelI=Iabc  Ipu=off  Pbase=100e6  Vbase=400/sqrt(2)  OutputType=Complex  PhasorSimulation=off  PSBequivalent=0
  A : PMIOPort  Side=Left
  B : PMIOPort  Port=2  Side=Left
  C : PMIOPort  Port=3  Side=Left
  "N " : PMIOPort  Tag=PMCPort  Port=4  Side=Left
  a : PMIOPort  Tag=PMCPort  Port=5  Side=Right
  b : PMIOPort  Tag=PMCPort  Port=6  Side=Right
  c : PMIOPort  Tag=PMCPort  Port=7  Side=Right
  n : PMIOPort  Tag=PMCPort  Port=8  Side=Right
  V_out : Outport
  tag scope: Vabc_B7=global
  wires:
  Three-Phase V-I Measurement/1 -> RMS/1
  RMS/1 -> MATLAB Function/1(u)
  MATLAB Function/1(y) -> [Vabc_B7], V_out/1
  connections:
  A/RConn1 -- Three-Phase V-I Measurement/LConn1
  B/RConn1 -- Three-Phase V-I Measurement/LConn2
  C/RConn1 -- Three-Phase V-I Measurement/LConn3
  a/RConn1 -- Three-Phase V-I Measurement/RConn1
  b/RConn1 -- Three-Phase V-I Measurement/RConn2
  c/RConn1 -- Three-Phase V-I Measurement/RConn3
  n/RConn1 -- "N "/RConn1

== system LV_grid/B8 ==
  MATLAB Function : MATLAB Function  TreatAsAtomicUnit=on
  RMS : spsRMSLib/RMS  TrueRMS=on  Freq=50  RMSInit=1  Ts=5e-4
  Three-Phase V-I Measurement : spsThreePhaseVIMeasurementLib/Three-Phase V-I Measurement  VoltageMeasurement=phase-to-ground  SetLabelV=off  LabelV=Vabc_B1  Vpu=on  VpuLL=off  CurrentMeasurement=no  SetLabelI=off  LabelI=Iabc  Ipu=off  Pbase=100e6  Vbase=400/sqrt(2)  OutputType=Complex  PhasorSimulation=off  PSBequivalent=0
  A : PMIOPort  Side=Left
  B : PMIOPort  Port=2  Side=Left
  C : PMIOPort  Port=3  Side=Left
  "N " : PMIOPort  Tag=PMCPort  Port=4  Side=Left
  a : PMIOPort  Tag=PMCPort  Port=5  Side=Right
  b : PMIOPort  Tag=PMCPort  Port=6  Side=Right
  c : PMIOPort  Tag=PMCPort  Port=7  Side=Right
  n : PMIOPort  Tag=PMCPort  Port=8  Side=Right
  V_out : Outport
  tag scope: Vabc_B8=global
  wires:
  Three-Phase V-I Measurement/1 -> RMS/1
  RMS/1 -> MATLAB Function/1(u)
  MATLAB Function/1(y) -> [Vabc_B8], V_out/1
  connections:
  A/RConn1 -- Three-Phase V-I Measurement/LConn1
  B/RConn1 -- Three-Phase V-I Measurement/LConn2
  C/RConn1 -- Three-Phase V-I Measurement/LConn3
  a/RConn1 -- Three-Phase V-I Measurement/RConn1
  b/RConn1 -- Three-Phase V-I Measurement/RConn2
  c/RConn1 -- Three-Phase V-I Measurement/RConn3
  n/RConn1 -- "N "/RConn1

== system LV_grid/B9 ==
  MATLAB Function : MATLAB Function  TreatAsAtomicUnit=on
  RMS : spsRMSLib/RMS  TrueRMS=on  Freq=50  RMSInit=1  Ts=5e-4
  Three-Phase V-I Measurement : spsThreePhaseVIMeasurementLib/Three-Phase V-I Measurement  VoltageMeasurement=phase-to-ground  SetLabelV=off  LabelV=Vabc_B1  Vpu=on  VpuLL=off  CurrentMeasurement=no  SetLabelI=off  LabelI=Iabc  Ipu=off  Pbase=100e6  Vbase=400/sqrt(2)  OutputType=Complex  PhasorSimulation=off  PSBequivalent=0
  A : PMIOPort  Side=Left
  B : PMIOPort  Port=2  Side=Left
  C : PMIOPort  Port=3  Side=Left
  "N " : PMIOPort  Tag=PMCPort  Port=4  Side=Left
  a : PMIOPort  Tag=PMCPort  Port=5  Side=Right
  b : PMIOPort  Tag=PMCPort  Port=6  Side=Right
  c : PMIOPort  Tag=PMCPort  Port=7  Side=Right
  n : PMIOPort  Tag=PMCPort  Port=8  Side=Right
  V_out : Outport
  tag scope: Vabc_B9=global
  wires:
  Three-Phase V-I Measurement/1 -> RMS/1
  RMS/1 -> MATLAB Function/1(u)
  MATLAB Function/1(y) -> [Vabc_B9], V_out/1
  connections:
  A/RConn1 -- Three-Phase V-I Measurement/LConn1
  B/RConn1 -- Three-Phase V-I Measurement/LConn2
  C/RConn1 -- Three-Phase V-I Measurement/LConn3
  a/RConn1 -- Three-Phase V-I Measurement/RConn1
  b/RConn1 -- Three-Phase V-I Measurement/RConn2
  c/RConn1 -- Three-Phase V-I Measurement/RConn3
  n/RConn1 -- "N "/RConn1

== system LV_grid/L1 ==
  note: 2.5m
  L1 : Subsystem
  A : PMIOPort  Side=Left
  B : PMIOPort  Port=2  Side=Left
  C : PMIOPort  Port=3  Side=Left
  N : PMIOPort  Port=4  Side=Left
  a : PMIOPort  Port=5  Side=Right
  b : PMIOPort  Port=6  Side=Right
  c : PMIOPort  Port=7  Side=Right
  n : PMIOPort  Port=8  Side=Right
  connections:
  n/RConn1 -- L1/RConn4
  L1/LConn4 -- N/RConn1
  L1/LConn3 -- C/RConn1
  L1/LConn2 -- B/RConn1
  L1/LConn1 -- A/RConn1
  L1/RConn1 -- a/RConn1
  L1/RConn2 -- b/RConn1
  L1/RConn3 -- c/RConn1

== system LV_grid/L10 ==
  note: 2.5m
  note: 2.5m
  Ground : spsGroundLib/Ground  LConnTagsString=a
  L1 : Subsystem
  L2 : Subsystem
  A : PMIOPort  Side=Left
  B : PMIOPort  Port=2  Side=Left
  C : PMIOPort  Port=3  Side=Left
  N : PMIOPort  Port=4  Side=Left
  a : PMIOPort  Port=5  Side=Right
  b : PMIOPort  Port=6  Side=Right
  c : PMIOPort  Port=7  Side=Right
  n : PMIOPort  Port=8  Side=Right
  connections:
  L2/RConn4 -- n/RConn1
  L1/RConn4 -- L2/LConn4 -- Ground/LConn1
  L1/LConn4 -- N/RConn1
  L1/LConn3 -- C/RConn1
  L1/LConn2 -- B/RConn1
  L1/LConn1 -- A/RConn1
  L2/LConn1 -- L1/RConn1
  L2/LConn2 -- L1/RConn2
  L2/LConn3 -- L1/RConn3
  L2/RConn1 -- a/RConn1
  L2/RConn2 -- b/RConn1
  L2/RConn3 -- c/RConn1

== system LV_grid/L11 ==
  note: 2.5m
  note: 2.5m
  Ground : spsGroundLib/Ground  LConnTagsString=a
  L1 : Subsystem
  L2 : Subsystem
  A : PMIOPort  Side=Left
  B : PMIOPort  Port=2  Side=Left
  C : PMIOPort  Port=3  Side=Left
  N : PMIOPort  Port=4  Side=Left
  a : PMIOPort  Port=5  Side=Right
  b : PMIOPort  Port=6  Side=Right
  c : PMIOPort  Port=7  Side=Right
  n : PMIOPort  Port=8  Side=Right
  connections:
  L2/RConn4 -- n/RConn1
  L1/RConn4 -- L2/LConn4 -- Ground/LConn1
  L1/LConn4 -- N/RConn1
  L1/LConn3 -- C/RConn1
  L1/LConn2 -- B/RConn1
  L1/LConn1 -- A/RConn1
  L2/LConn1 -- L1/RConn1
  L2/LConn2 -- L1/RConn2
  L2/LConn3 -- L1/RConn3
  L2/RConn1 -- a/RConn1
  L2/RConn2 -- b/RConn1
  L2/RConn3 -- c/RConn1

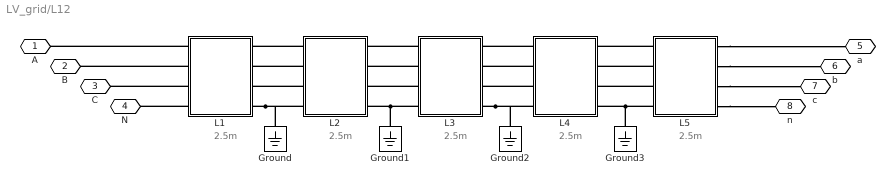
== system LV_grid/L12 ==
  note: 2.5m
  note: 2.5m
  note: 2.5m
  note: 2.5m
  note: 2.5m
  Ground{,1..3} (4 alike) : spsGroundLib/Ground  LConnTagsString=a
  L1 : Subsystem
  L2 : Subsystem
  L3 : Subsystem
  L4 : Subsystem
  L5 : Subsystem
  A : PMIOPort  Side=Left
  B : PMIOPort  Port=2  Side=Left
  C : PMIOPort  Port=3  Side=Left
  N : PMIOPort  Port=4  Side=Left
  a : PMIOPort  Port=5  Side=Right
  b : PMIOPort  Port=6  Side=Right
  c : PMIOPort  Port=7  Side=Right
  n : PMIOPort  Port=8  Side=Right
  connections:
  L1/LConn1 -- A/RConn1
  L1/LConn4 -- N/RConn1
  L1/LConn2 -- B/RConn1
  L1/LConn3 -- C/RConn1
  L5/LConn4 -- L4/RConn4 -- Ground3/LConn1
  L3/RConn4 -- L4/LConn4 -- Ground2/LConn1
  L5/RConn4 -- n/RConn1
  L3/LConn4 -- L2/RConn4 -- Ground1/LConn1
  L1/RConn4 -- L2/LConn4 -- Ground/LConn1
  L5/LConn1 -- L4/RConn1
  L5/LConn2 -- L4/RConn2
  L5/LConn3 -- L4/RConn3
  L3/LConn1 -- L2/RConn1
  L3/LConn2 -- L2/RConn2
  L3/LConn3 -- L2/RConn3
  L5/RConn1 -- a/RConn1
  L5/RConn2 -- b/RConn1
  L5/RConn3 -- c/RConn1
  L2/LConn1 -- L1/RConn1
  L2/LConn2 -- L1/RConn2
  L2/LConn3 -- L1/RConn3
  L4/LConn1 -- L3/RConn1
  L4/LConn2 -- L3/RConn2
  L4/LConn3 -- L3/RConn3

== system LV_grid/L13 ==
  note: 2.5m
  note: 2.5m
  Ground : spsGroundLib/Ground  LConnTagsString=a
  L1 : Subsystem
  L2 : Subsystem
  A : PMIOPort  Side=Left
  B : PMIOPort  Port=2  Side=Left
  C : PMIOPort  Port=3  Side=Left
  N : PMIOPort  Port=4  Side=Left
  a : PMIOPort  Port=5  Side=Right
  b : PMIOPort  Port=6  Side=Right
  c : PMIOPort  Port=7  Side=Right
  n : PMIOPort  Port=8  Side=Right
  connections:
  L2/RConn4 -- n/RConn1
  L1/RConn4 -- L2/LConn4 -- Ground/LConn1
  L1/LConn4 -- N/RConn1
  L1/LConn3 -- C/RConn1
  L1/LConn2 -- B/RConn1
  L1/LConn1 -- A/RConn1
  L2/RConn1 -- a/RConn1
  L2/RConn2 -- b/RConn1
  L2/RConn3 -- c/RConn1
  L2/LConn1 -- L1/RConn1
  L2/LConn2 -- L1/RConn2
  L2/LConn3 -- L1/RConn3

== system LV_grid/L14 ==
  note: 2.5m
  L1 : Subsystem
  A : PMIOPort  Side=Left
  B : PMIOPort  Port=2  Side=Left
  C : PMIOPort  Port=3  Side=Left
  N : PMIOPort  Port=4  Side=Left
  a : PMIOPort  Port=5  Side=Right
  b : PMIOPort  Port=6  Side=Right
  c : PMIOPort  Port=7  Side=Right
  n : PMIOPort  Port=8  Side=Right
  connections:
  B/RConn1 -- L1/LConn2
  n/RConn1 -- L1/RConn4
  C/RConn1 -- L1/LConn3
  N/RConn1 -- L1/LConn4
  A/RConn1 -- L1/LConn1
  L1/RConn1 -- a/RConn1
  L1/RConn2 -- b/RConn1
  L1/RConn3 -- c/RConn1

== system LV_grid/L15 ==
  note: 2.5m
  note: 2.5m
  Ground : spsGroundLib/Ground  LConnTagsString=a
  L1 : Subsystem
  L2 : Subsystem
  A : PMIOPort  Side=Left
  B : PMIOPort  Port=2  Side=Left
  C : PMIOPort  Port=3  Side=Left
  N : PMIOPort  Port=4  Side=Left
  a : PMIOPort  Port=5  Side=Right
  b : PMIOPort  Port=6  Side=Right
  c : PMIOPort  Port=7  Side=Right
  n : PMIOPort  Port=8  Side=Right
  connections:
  L2/RConn4 -- n/RConn1
  L1/RConn4 -- L2/LConn4 -- Ground/LConn1
  L1/LConn4 -- N/RConn1
  L1/LConn3 -- C/RConn1
  L1/LConn2 -- B/RConn1
  L1/LConn1 -- A/RConn1
  L2/LConn1 -- L1/RConn1
  L2/LConn2 -- L1/RConn2
  L2/LConn3 -- L1/RConn3
  L2/RConn1 -- a/RConn1
  L2/RConn2 -- b/RConn1
  L2/RConn3 -- c/RConn1

== system LV_grid/L16 ==
  note: 2.5m
  L1 : Subsystem
  A : PMIOPort  Side=Left
  B : PMIOPort  Port=2  Side=Left
  C : PMIOPort  Port=3  Side=Left
  N : PMIOPort  Port=4  Side=Left
  a : PMIOPort  Port=5  Side=Right
  b : PMIOPort  Port=6  Side=Right
  c : PMIOPort  Port=7  Side=Right
  n : PMIOPort  Port=8  Side=Right
  connections:
  B/RConn1 -- L1/LConn2
  n/RConn1 -- L1/RConn4
  C/RConn1 -- L1/LConn3
  N/RConn1 -- L1/LConn4
  A/RConn1 -- L1/LConn1
  L1/RConn1 -- a/RConn1
  L1/RConn2 -- b/RConn1
  L1/RConn3 -- c/RConn1

== system LV_grid/L17 ==
  note: 2.5m
  note: 2.5m
  note: 2.5m
  Ground : spsGroundLib/Ground  LConnTagsString=a
  Ground1 : spsGroundLib/Ground  LConnTagsString=a
  L1 : Subsystem
  L2 : Subsystem
  L3 : Subsystem
  A : PMIOPort  Side=Left
  B : PMIOPort  Port=2  Side=Left
  C : PMIOPort  Port=3  Side=Left
  N : PMIOPort  Port=4  Side=Left
  a : PMIOPort  Port=5  Side=Right
  b : PMIOPort  Port=6  Side=Right
  c : PMIOPort  Port=7  Side=Right
  n : PMIOPort  Port=8  Side=Right
  connections:
  L1/LConn2 -- B/RConn1
  L1/LConn4 -- N/RConn1
  L1/LConn1 -- A/RConn1
  L1/RConn4 -- L2/LConn4 -- Ground/LConn1
  L1/LConn3 -- C/RConn1
  L3/RConn4 -- n/RConn1
  L2/RConn4 -- L3/LConn4 -- Ground1/LConn1
  L3/RConn1 -- a/RConn1
  L3/RConn2 -- b/RConn1
  L3/RConn3 -- c/RConn1
  L3/LConn1 -- L2/RConn1
  L3/LConn2 -- L2/RConn2
  L3/LConn3 -- L2/RConn3
  L2/LConn1 -- L1/RConn1
  L2/LConn2 -- L1/RConn2
  L2/LConn3 -- L1/RConn3

== system LV_grid/L18 ==
  note: 2.5m
  note: 2.5m
  Ground : spsGroundLib/Ground  LConnTagsString=a
  L1 : Subsystem
  L2 : Subsystem
  A : PMIOPort  Side=Left
  B : PMIOPort  Port=2  Side=Left
  C : PMIOPort  Port=3  Side=Left
  N : PMIOPort  Port=4  Side=Left
  a : PMIOPort  Port=5  Side=Right
  b : PMIOPort  Port=6  Side=Right
  c : PMIOPort  Port=7  Side=Right
  n : PMIOPort  Port=8  Side=Right
  connections:
  L2/RConn4 -- n/RConn1
  L1/RConn4 -- L2/LConn4 -- Ground/LConn1
  L1/LConn4 -- N/RConn1
  L1/LConn3 -- C/RConn1
  L1/LConn2 -- B/RConn1
  L1/LConn1 -- A/RConn1
  L2/LConn1 -- L1/RConn1
  L2/LConn2 -- L1/RConn2
  L2/LConn3 -- L1/RConn3
  L2/RConn1 -- a/RConn1
  L2/RConn2 -- b/RConn1
  L2/RConn3 -- c/RConn1

== system LV_grid/L19 ==
  note: 2.5m
  L1 : Subsystem
  A : PMIOPort  Side=Left
  B : PMIOPort  Port=2  Side=Left
  C : PMIOPort  Port=3  Side=Left
  N : PMIOPort  Port=4  Side=Left
  a : PMIOPort  Port=5  Side=Right
  b : PMIOPort  Port=6  Side=Right
  c : PMIOPort  Port=7  Side=Right
  n : PMIOPort  Port=8  Side=Right
  connections:
  B/RConn1 -- L1/LConn2
  n/RConn1 -- L1/RConn4
  C/RConn1 -- L1/LConn3
  N/RConn1 -- L1/LConn4
  A/RConn1 -- L1/LConn1
  L1/RConn1 -- a/RConn1
  L1/RConn2 -- b/RConn1
  L1/RConn3 -- c/RConn1

== system LV_grid/L2 ==
  note: 2.5m
  L1 : Subsystem
  A : PMIOPort  Side=Left
  B : PMIOPort  Port=2  Side=Left
  C : PMIOPort  Port=3  Side=Left
  N : PMIOPort  Port=4  Side=Left
  a : PMIOPort  Port=5  Side=Right
  b : PMIOPort  Port=6  Side=Right
  c : PMIOPort  Port=7  Side=Right
  n : PMIOPort  Port=8  Side=Right
  connections:
  B/RConn1 -- L1/LConn2
  n/RConn1 -- L1/RConn4
  C/RConn1 -- L1/LConn3
  N/RConn1 -- L1/LConn4
  A/RConn1 -- L1/LConn1
  L1/RConn1 -- a/RConn1
  L1/RConn2 -- b/RConn1
  L1/RConn3 -- c/RConn1

== system LV_grid/L20 ==
  note: 2.5m
  note: 2.5m
  note: 2.5m
  Ground : spsGroundLib/Ground  LConnTagsString=a
  Ground1 : spsGroundLib/Ground  LConnTagsString=a
  L1 : Subsystem
  L2 : Subsystem
  L3 : Subsystem
  A : PMIOPort  Side=Left
  B : PMIOPort  Port=2  Side=Left
  C : PMIOPort  Port=3  Side=Left
  N : PMIOPort  Port=4  Side=Left
  a : PMIOPort  Port=5  Side=Right
  b : PMIOPort  Port=6  Side=Right
  c : PMIOPort  Port=7  Side=Right
  n : PMIOPort  Port=8  Side=Right
  connections:
  L1/LConn2 -- B/RConn1
  L1/LConn4 -- N/RConn1
  L1/LConn1 -- A/RConn1
  L1/RConn4 -- L2/LConn4 -- Ground/LConn1
  L1/LConn3 -- C/RConn1
  L3/RConn4 -- n/RConn1
  L2/RConn4 -- L3/LConn4 -- Ground1/LConn1
  L3/RConn1 -- a/RConn1
  L3/RConn2 -- b/RConn1
  L3/RConn3 -- c/RConn1
  L2/LConn1 -- L1/RConn1
  L2/LConn2 -- L1/RConn2
  L2/LConn3 -- L1/RConn3
  L3/LConn1 -- L2/RConn1
  L3/LConn2 -- L2/RConn2
  L3/LConn3 -- L2/RConn3

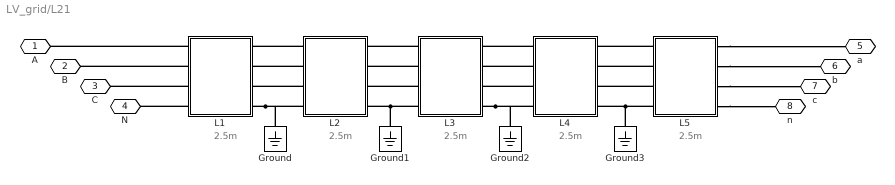
== system LV_grid/L21 ==
  note: 2.5m
  note: 2.5m
  note: 2.5m
  note: 2.5m
  note: 2.5m
  Ground{,1..3} (4 alike) : spsGroundLib/Ground  LConnTagsString=a
  L1 : Subsystem
  L2 : Subsystem
  L3 : Subsystem
  L4 : Subsystem
  L5 : Subsystem
  A : PMIOPort  Side=Left
  B : PMIOPort  Port=2  Side=Left
  C : PMIOPort  Port=3  Side=Left
  N : PMIOPort  Port=4  Side=Left
  a : PMIOPort  Port=5  Side=Right
  b : PMIOPort  Port=6  Side=Right
  c : PMIOPort  Port=7  Side=Right
  n : PMIOPort  Port=8  Side=Right
  connections:
  L1/LConn1 -- A/RConn1
  L1/LConn4 -- N/RConn1
  L1/LConn2 -- B/RConn1
  L1/LConn3 -- C/RConn1
  L5/LConn4 -- L4/RConn4 -- Ground3/LConn1
  L3/RConn4 -- L4/LConn4 -- Ground2/LConn1
  L5/RConn4 -- n/RConn1
  L3/LConn4 -- L2/RConn4 -- Ground1/LConn1
  L1/RConn4 -- L2/LConn4 -- Ground/LConn1
  L5/RConn1 -- a/RConn1
  L5/RConn2 -- b/RConn1
  L5/RConn3 -- c/RConn1
  L2/LConn1 -- L1/RConn1
  L2/LConn2 -- L1/RConn2
  L2/LConn3 -- L1/RConn3
  L4/LConn1 -- L3/RConn1
  L4/LConn2 -- L3/RConn2
  L4/LConn3 -- L3/RConn3
  L5/LConn1 -- L4/RConn1
  L5/LConn2 -- L4/RConn2
  L5/LConn3 -- L4/RConn3
  L3/LConn1 -- L2/RConn1
  L3/LConn2 -- L2/RConn2
  L3/LConn3 -- L2/RConn3

== system LV_grid/L22 ==
  note: 2.5m
  note: 2.5m
  Ground : spsGroundLib/Ground  LConnTagsString=a
  L1 : Subsystem
  L2 : Subsystem
  A : PMIOPort  Side=Left
  B : PMIOPort  Port=2  Side=Left
  C : PMIOPort  Port=3  Side=Left
  N : PMIOPort  Port=4  Side=Left
  a : PMIOPort  Port=5  Side=Right
  b : PMIOPort  Port=6  Side=Right
  c : PMIOPort  Port=7  Side=Right
  n : PMIOPort  Port=8  Side=Right
  connections:
  L2/RConn4 -- n/RConn1
  L1/RConn4 -- L2/LConn4 -- Ground/LConn1
  L1/LConn4 -- N/RConn1
  L1/LConn3 -- C/RConn1
  L1/LConn2 -- B/RConn1
  L1/LConn1 -- A/RConn1
  L2/RConn1 -- a/RConn1
  L2/RConn2 -- b/RConn1
  L2/RConn3 -- c/RConn1
  L2/LConn1 -- L1/RConn1
  L2/LConn2 -- L1/RConn2
  L2/LConn3 -- L1/RConn3

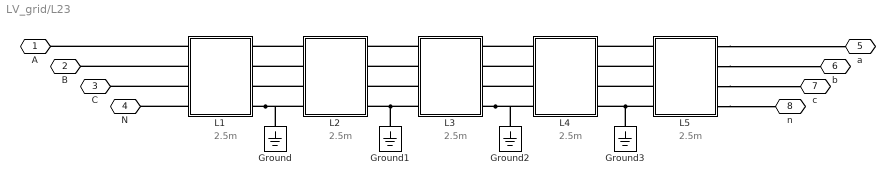
== system LV_grid/L23 ==
  note: 2.5m
  note: 2.5m
  note: 2.5m
  note: 2.5m
  note: 2.5m
  Ground{,1..3} (4 alike) : spsGroundLib/Ground  LConnTagsString=a
  L1 : Subsystem
  L2 : Subsystem
  L3 : Subsystem
  L4 : Subsystem
  L5 : Subsystem
  A : PMIOPort  Side=Left
  B : PMIOPort  Port=2  Side=Left
  C : PMIOPort  Port=3  Side=Left
  N : PMIOPort  Port=4  Side=Left
  a : PMIOPort  Port=5  Side=Right
  b : PMIOPort  Port=6  Side=Right
  c : PMIOPort  Port=7  Side=Right
  n : PMIOPort  Port=8  Side=Right
  connections:
  L1/LConn1 -- A/RConn1
  L1/LConn4 -- N/RConn1
  L1/LConn2 -- B/RConn1
  L1/LConn3 -- C/RConn1
  L5/LConn4 -- L4/RConn4 -- Ground3/LConn1
  L3/RConn4 -- L4/LConn4 -- Ground2/LConn1
  L5/RConn4 -- n/RConn1
  L3/LConn4 -- L2/RConn4 -- Ground1/LConn1
  L1/RConn4 -- L2/LConn4 -- Ground/LConn1
  L4/LConn1 -- L3/RConn1
  L4/LConn2 -- L3/RConn2
  L4/LConn3 -- L3/RConn3
  L2/LConn1 -- L1/RConn1
  L2/LConn2 -- L1/RConn2
  L2/LConn3 -- L1/RConn3
  L5/RConn1 -- a/RConn1
  L5/RConn2 -- b/RConn1
  L5/RConn3 -- c/RConn1
  L5/LConn1 -- L4/RConn1
  L5/LConn2 -- L4/RConn2
  L5/LConn3 -- L4/RConn3
  L3/LConn1 -- L2/RConn1
  L3/LConn2 -- L2/RConn2
  L3/LConn3 -- L2/RConn3

== system LV_grid/L24 ==
  note: 2.5m
  note: 2.5m
  note: 2.5m
  note: 2.5m
  Ground : spsGroundLib/Ground  LConnTagsString=a
  Ground1 : spsGroundLib/Ground  LConnTagsString=a
  Ground2 : spsGroundLib/Ground  LConnTagsString=a
  L1 : Subsystem
  L2 : Subsystem
  L3 : Subsystem
  L4 : Subsystem
  A : PMIOPort  Side=Left
  B : PMIOPort  Port=2  Side=Left
  C : PMIOPort  Port=3  Side=Left
  N : PMIOPort  Port=4  Side=Left
  a : PMIOPort  Port=5  Side=Right
  b : PMIOPort  Port=6  Side=Right
  c : PMIOPort  Port=7  Side=Right
  n : PMIOPort  Port=8  Side=Right
  connections:
  L1/LConn3 -- C/RConn1
  L2/RConn4 -- L3/LConn4 -- Ground1/LConn1
  L1/LConn4 -- N/RConn1
  L1/LConn2 -- B/RConn1
  L1/LConn1 -- A/RConn1
  L1/RConn4 -- L2/LConn4 -- Ground/LConn1
  L3/RConn4 -- L4/LConn4 -- Ground2/LConn1
  L4/RConn4 -- n/RConn1
  L4/RConn1 -- a/RConn1
  L4/RConn2 -- b/RConn1
  L4/RConn3 -- c/RConn1
  L3/LConn1 -- L2/RConn1
  L3/LConn2 -- L2/RConn2
  L3/LConn3 -- L2/RConn3
  L2/LConn1 -- L1/RConn1
  L2/LConn2 -- L1/RConn2
  L2/LConn3 -- L1/RConn3
  L4/LConn1 -- L3/RConn1
  L4/LConn2 -- L3/RConn2
  L4/LConn3 -- L3/RConn3
